simulink model "CSTD1_OpenLoopModel"  (Simulink 10.1)
settings: Solver=ode3  StartTime=0.0  StopTime=2  FixedStep=0.001  RelTol=1e-3  EnableMultiTasking=on
InitFcn:
  | load state_space_model.mat;
undefined symbols (not defined in the file or in its folder): A_sim, B_sim, C_sim, D_sim
libraries: simulink x2
settings Model: Creator=jb  LastModifiedBy=nwegy
settings DataIOCC: LimitDataPoints=on  SignalLoggingSaveFormat=ModelDataLogs
settings OptimizationCC: ExpressionDepthLimit=2147483647
settings DebuggingCC: SolverPrmCheckMsg=warning  FcnCallInpInsideContextMsg=warning  StateNameClashWarn=warning
settings ConfigComp: CovSFcnEnable=off

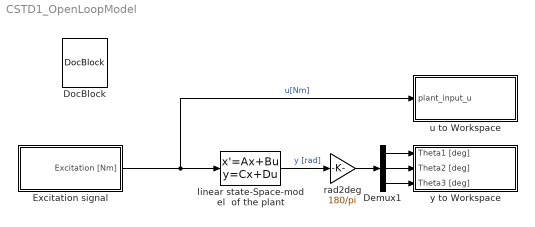
== system CSTD1_OpenLoopModel ==
  Demux1 : Demux  Outputs=3
  DocBlock : simulink/Model-Wide Utilities/DocBlock  DocumentType=Text
  Excitation signal : Subsystem
  linear state-Space-model  of the plant : StateSpace  A=A_sim  B=B_sim  C=C_sim  D=D_sim  InitialCondition=0
  rad2deg : Gain  Gain=180/pi
  u to Workspace : Subsystem
  y to Workspace : Subsystem
  wires:
  Excitation signal/1(Excitation [Nm]) -> linear state-Space-model  of the plant/1, u to Workspace/1(plant_input_u)  "u[Nm]"
  linear state-Space-model  of the plant/1 -> rad2deg/1  "y [rad]"
  Demux1/1 -> y to Workspace/1(Theta1 [deg])
  Demux1/2 -> y to Workspace/2(Theta2 [deg])
  Demux1/3 -> y to Workspace/3(Theta3 [deg])
  rad2deg/1 -> Demux1/1

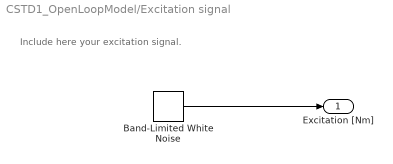
== system CSTD1_OpenLoopModel/Excitation signal ==
  note: Include here your excitation signal.
  Band-Limited White Noise : simulink/Sources/Band-Limited White Noise  Cov=[0.000194]  Ts=0.001  seed=[23341]
  Excitation [Nm] : Outport  VectorParamsAs1DForOutWhenUnconnected=off
  wires:
  Band-Limited White Noise/1 -> Excitation [Nm]/1

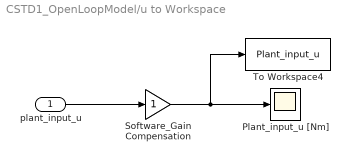
== system CSTD1_OpenLoopModel/u to Workspace ==
  plant_input_u : Inport
  Plant_input_u [Nm] : Scope
  Software_Gain Compensation : Gain
  To Workspace4 : ToWorkspace  VariableName=Plant_input_u  SampleTime=-1
  wires:
  Software_Gain Compensation/1 -> Plant_input_u [Nm]/1, To Workspace4/1
  plant_input_u/1 -> Software_Gain Compensation/1

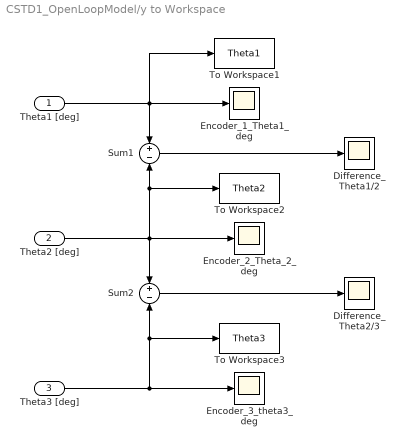
== system CSTD1_OpenLoopModel/y to Workspace ==
  Theta1 [deg] : Inport
  Theta2 [deg] : Inport  Port=2
  Theta3 [deg] : Inport  Port=3
  Difference_Theta1/2 : Scope
  Difference_Theta2/3 : Scope
  Encoder_1_Theta1_deg : Scope
  Encoder_2_Theta_2_deg : Scope
  Encoder_3_theta3_deg : Scope
  Sum1 : Sum  Inputs=+-
  Sum2 : Sum  Inputs=+-
  To Workspace1 : ToWorkspace  VariableName=Theta1  SampleTime=-1
  To Workspace2 : ToWorkspace  VariableName=Theta2  SampleTime=-1
  To Workspace3 : ToWorkspace  VariableName=Theta3  SampleTime=-1
  wires:
  Theta1 [deg]/1 -> Encoder_1_Theta1_deg/1, Sum1/1, To Workspace1/1
  Theta3 [deg]/1 -> Encoder_3_theta3_deg/1, Sum2/2, To Workspace3/1
  Sum1/1 -> Difference_Theta1/2/1
  Sum2/1 -> Difference_Theta2/3/1
  Theta2 [deg]/1 -> To Workspace2/1, Sum1/2, Encoder_2_Theta_2_deg/1, Sum2/1
